simulink model "GFM_NN_closedloop"  (R2025a)
settings: Solver=FixedStepAuto  StartTime=0.0  StopTime=8  FixedStep=1e-6  RelTol=1e-5
PostLoadFcn:
  | , if any(exist('dsrtsu_mdlpostloadfcn', 'file') == [2, 3, 6]), try dsrtsu_mdlpostloadfcn('Execute', bdroot); catch fprintf('Error in PostLoadFcn (dsrtsu_mdlpostloadfcn) for model "%s":\n %s\n', bdroot, lasterr); end, end,
InitFcn:
  | %% ---------sampling time---------
  | fs=10000;
  | Ts = 1/fs; % 1/fs = sampling period;
  | Tsp=Ts;
  | ws=2*pi*fs;
  | Tc = Ts/1;
  | Tch = inf;
  | % Interrupt shift
  | %Tint=0.25e-6;
  | Tint=0.25e-6;
  | %Tint=0;
  | 
  | %% Frequency
  | fsw = 10e3;
  | Tsp = 1 / fsw;
  | % Ts = 1e-6;
  | 
  | %% Grid parameters
  | Vg_LG_RMS = 110;
  | Vg_LL_RMS = Vg_LG_RMS * sqrt(3);
  | f1 = 50;
  | w1 = f1 * 2 * pi;
  | 
  | Lg = 15e-3;
  | Rg = w1 * Lg * 0.05;
  | 
  | %% GFM converter
  | peak_phase_to_earth = sqrt(2)/sqrt(3);
  | SN_GFM = 4e3;
  | PN_GFM = SN_GFM;
  | Vtr_1 = 132;
  | V_base_GFL = Vtr_1*peak_phase_to_earth;
  | I_base_GFL = SN_GFM*peak_phase_to_earth/Vtr_1;
  | 
  | Vs_LL_RMS = Vg_LL_RMS;
  | VDC = 600;
  | 
  | Ls = 3e-3;
  | Rs = w1 * Ls * 0.05;
  | % Rs = 1e-1;
  | Cf = 10e-6;
  | Rf = 1e-3;
  | % Rf = 1;
  | 
  | %% Base values
  | w_Base = 1;
  | %w_Base = 2*pi*f1;
  | V_Base_GFM = sqrt(2) * Vs_LL_RMS / sqrt(3);      % Peak value
  | S_Base_GFM = SN_GFM;
  | I_Base_GFM = sqrt(2) * (S_Base_GFM / 3) / (V_Base_GFM / sqrt(2));     % Peak value
  | Z_Base_GFM = V_Base_GFM / I_Base_GFM;
  | L_Base_GFM = Z_Base_GFM / w_Base;
  | C_Base_GFM = 1 / (w_Base * Z_Base_GFM);
  | 
  | w1_pu = w1 / w_Base;
  | 
  | %% PU values
  | Ls * w1_pu / Z_Base_GFM
  | Ls_pu = Ls / Z_Base_GFM;
  | Lg_pu = Lg / Z_Base_GFM;
  | SCR = 1 / (Lg * w1_pu / Z_Base_GFM)
  | 
  | %% PLL parameters
  | %Kp_PLL = 327.1; %654.3; %32.7;
  | Ki_PLL = 1/0.000013; %1/0.00000325; %1/0.0013;
  | 
  | Kp_SYC = 2;
  | Ki_SYC = 5;
  | 
  | Kp_PQ = 0.1;
  | Ki_PQ = 0.4;
  | 
  | % Kpcc = 5;
  | Kicc = 1/0.01;
  | 
  | %% LPF parameters
  | wp = 2 * pi * 100;
  | wq = 2 * pi * 100;
  | wv = 2 * pi * 100;
  | 
  | %% GFM parameters
  | Pref = 1;
  | kPi = 0.05 * w1_pu;
  | Ra = 0.1;
  | wR = 0.1 * w1_pu;
  | wI = 10 * w1_pu;
  | 
  | kV = 20;
  | kQ = 0.1;
  | 
  | %% Discretization of decoupling
  | s = tf('s');
  | 
  | RV = (Ra*s)/(s+wR);
  | % RV = RV*(wI)/(s+wI);
  | 
  | R1d = c2d(RV , Tsp , 'tustin');
  | dR1num = R1d.Numerator{1};
  | dR1den = R1d.Denominator{1};
  | 
  | %% Discretization of active damping
  | wlpf = 2 * pi * 100;
  | G1st = wlpf / (s + wlpf);
  | G2nd = G1st * G1st;
  | Gc = s * G2nd;
  | Gcd = c2d(Gc , Tsp , 'tustin');
  | 
  | Gcdnum = Gcd.Numerator{1};
  | Gcdden = Gcd.Denominator{1};
  | 
  | %ADC
  | UdcTransdRatio = 25e-3/800;
  | UcaTransdRatio = 25e-3/600;
  | UcbTransdRatio = 25e-3/600;
  | UccTransdRatio = 25e-3/600;
  | UgaTransdRatio = 25e-3/400;
  | UgbTransdRatio = 25e-3/400;
  | UgcTransdRatio = 25e-3/400;
  | 
  | RMeasIa = 220;
  | RMeasIb = 220;
  | RMeasIc = 220;
  | RMeasIdc = 215;
  | RMeasUdc = 237;
  | RMeasUa = 220;
  | RMeasUb = 220;
  | RMeasUc = 220;
  | 
  | LemTurnsIa = 2;
  | LemTurnsIb = 2;
  | LemTurnsIc = 2;
  | 
  | LemTurnsIa1 = 4;
  | LemTurnsIb1 = 4;
  | LemTurnsIc1 = 4;
  | 
  | IaTransdRatio = LemTurnsIa/1000;
  | IbTransdRatio = LemTurnsIb/1000;
  | IcTransdRatio = LemTurnsIc/1000;
  | 
  | IaTransdRatio1 = LemTurnsIa1/1000;
  | IbTransdRatio1 = LemTurnsIb1/1000;
  | IcTransdRatio1 = LemTurnsIc1/1000;
  | 
  | %%
  | %% 1Hz--31Hz  per 1Hz
  | 
  | % degree =5;
  | % K =1;
  | % periods =600;
  | 
  | % PRBS = idinput((2^degree-1), 'prbs');
  | % PRBS = repmat(PRBS,periods + 1,1);
  | % PRBS = K*PRBS;
  | % PRBS_freq =31;
  | 
  | % t_vector=(1/PRBS_freq:1/PRBS_freq:length(PRBS)/PRBS_freq)';
  | % PRBS=[t_vector, PRBS];
  | % stop=t_vector(end);
  | 
  | 
  | %% ====================================================================================================================================================%%
  | %% 10Hz--310Hz  per 10Hz
  | 
  | % degree =5;
  | % K =1.5;
  | % periods =6000;
  | %
  | % PRBS = idinput((2^degree-1), 'prbs');
  | % PRBS = repmat(PRBS,periods + 1,1);
  | % PRBS = K*PRBS;
  | % PRBS_freq =310;
  | %
  | % t_vector=(1/PRBS_freq:1/PRBS_freq:length(PRBS)/PRBS_freq)';
  | % PRBS=[t_vector, PRBS];
  | % stop=t_vector(end);
  | 
  | 
  | %% ====================================================================================================================================================%%
  | %% 100Hz--3100Hz  per 100Hz
  | 
  | % degree =5;
  | % K =2;
  | % periods =10000;
  | %
  | % PRBS = idinput((2^degree-1), 'prbs');
  | % PRBS = repmat(PRBS,periods + 1,1);
  | % PRBS = K*PRBS;
  | % PRBS_freq =3100;
  | %
  | % t_vector=(1/PRBS_freq:1/PRBS_freq:length(PRBS)/PRBS_freq)';
  | % PRBS=[t_vector, PRBS];
  | % stop=t_vector(end);
  | %Kd=1;
  | %wL=0.3*ws;
  | 
  | %L1=4.5e-3;
  | %Tdel=1.5*Ts;
  | %PM=pi/4;%phase margin
  | %wc=(pi/2-PM)/Tdel;%magnitude crossover frequency
  | %Kp=wc*L1;%proportional gain
  | %Ki=wc*Kp/20;%fundamental integrator gain
model workspace (MAT data in the model file):
  W1 = [0.530351698399 -0.46726077795 -0.189978018403 0.581505596638 -0.976636350155 0.285457074642 -0.344555467367 -0.823834598064 0.260987460613 -0.174824804068 0.166140690446 -2.19062757492 ... (5120 elements, 64x80)]
  W2 = [0.0236483272165 -0.12587569654 -3.47338819504 -0.292541116476 -0.164569035172 -0.37011295557 -0.0788608714938 -0.34808665514 -0.0821482911706 0.0780714154243 -0.721733689308 -0.485419809818 ... (1024 elements, 16x64)]
  W3 = [-0.129827529192 0.112917125225 -0.211720749736 0.109386667609 -1.40702748299 -1.11484694481 -0.318361610174 0.218052342534 0.374470740557 -0.190498560667 -0.238774597645 0.996348917484 0.27190181613 -0.264939814806 -0.220842242241 0.382941007614]
  b1 = [-8.9806804657; -10.8322944641; 0.357735663652; -8.11319255829; -12.3089160919; -6.15159845352; -0.239361956716; -10.1425418854; -3.17705559731; -9.53854560852; -2.29398417473; -11.1701593399; -1.7048176527; -9.67482185364; -9.67645168304; -0.294388860464; -2.24801635742; -7.25962114334; -12.5521097183; -6.6342830658; -0.823176324368; 0.253660053015; -8.99686527252; -12.8170499802; -10.1545505524; -2.08569598198; -4.45409345627; -3.44555258751; -10.1237840652; -4.41725730896; -1.93720889091; -11.3758125305; -1.21599435806; -17.1822433472; -2.60073232651; -11.0052156448; -6.07818651199; -9.34351730347; -10.6377429962; 1.69822740555; -9.43974971771; -2.7141919136; -3.19006466866; -11.3538637161; -11.2651071548; -2.94875788689; -1.71119105816; -7.6843419075; -15.207570076; -0.106311887503; -10.9692764282; -0.920050501823; 0.828176736832; -11.2579984665; -9.09425544739; -7.6097574234; -0.587199747562; -5.53113889694; -2.76576495171; -1.6608453989; -10.8241662979; -8.84553050995; -0.99967366457; -11.8896923065]
  b2 = [-0.136206507683; -0.45766967535; -1.54362010956; -0.556495547295; -0.369174063206; -1.49981951714; -1.85871458054; -0.587826907635; -4.87963867188; -1.14077246189; -0.44449698925; -0.9487388134; 2.4190299511; 3.84015583992; -0.180305749178; -0.441644221544]
  b3 = 2.70423817635
  iqrValues = [999.929682567 999.948806394 999.974126382 1163.68199033 1249.86143465 1016.10909761 999.955656405 999.968539404 999.977085124 999.966554003 999.979581889 999.988183479 999.991575713 999.993056679 1000.02967135 1000.00803114 1000.0081017 1210.4487351 1499.93624967 1499.9370729 1406.48598833 937.760144727 1004.26905001 1026.06698255 1138.4066529 1206.84833926 1281.43314966 1372.93379822 1200.77275342 1298.83976016 1490.12450166 1497.42025213 1498.55627365 1498.83428777 1499.24135331 1499.39002656 1499.55488962 1499.65443504 1499.70746847 1499.73165249 1499.74454692 1499.76882354 1499.79135716 1499.80986709 1499.83281542 1499.8484425 1499.8654311 1499.87451238 1499.8928119 1499.9009956 1499.90976565 1499.91746661 1499.92756619 1499.93539792 1499.9414488 1499.94710313 1499.9507773 1499.95615869 1499.96087707 1499.96513792 1499.969596 1499.97293448 1499.97631403 1499.97913361 1499.98180466 1499.98376736 1499.9856365 1499.98732196 1499.98880177 1499.990067 1499.99120073 1499.9922432 1499.9932786 1499.99403762 1499.99470811 1499.99533602 1499.9958744 1499.99636227 1499.99677184 1499.99716187]
  medianValues = [1999.66013382 1999.76293028 1999.73262567 1999.76378275 1999.76361619 1999.77040731 1999.79192245 1999.85691047 1999.87382515 1999.88874694 1999.91524435 1999.91351393 1999.92374826 1999.91295141 1999.89897222 1999.91068089 1999.9210953 1999.9106703 1999.9196212 1999.92798731 1911.70708018 1395.87669838 1499.98470029 1499.98345327 1644.01690443 1805.89164886 1790.23759124 1810.28461467 1819.29782683 1874.70206922 1866.37458572 1829.46040718 1746.52407759 1689.08032976 1634.2809925 1690.42170061 1711.43926014 1714.57960898 1723.90792471 1755.22399993 1766.76731052 1745.61016029 1710.90545293 1744.81369568 1731.87842468 1711.49890061 1691.0235018 1685.21995546 1711.86371385 1706.17582468 1681.04912761 1670.10963643 1649.85367648 1649.94378709 1656.85502029 1681.84492812 1701.45866125 1703.86654039 1702.66606714 1701.58839466 1704.30441478 1719.94997721 1714.50309563 1724.69934828 1742.41991357 1753.39080321 1736.9800895 1742.57116721 1741.00321976 1748.99545485 1735.18183948 1717.61156426 1712.46451329 1713.44210291 1724.88072756 1740.57545678 1739.7916782 1723.53851422 1713.75990069 1700.06444303]
  mu = [-0.108593781339 -0.147308811259 -0.175534555128 -0.136585928467 -0.119784171193 -0.170883245612 -0.185899506459 -0.135931465846 -0.0891217813808 -0.0659545740614 -0.0558679902038 -0.052863332895 -0.0549410539837 -0.0621396876514 -0.0763691039853 -0.102015738859 -0.145826894941 -0.170573714468 -0.166261136131 -0.186454984398 -0.196618728586 -0.0474868984901 0.0493634627812 0.102614249626 0.0637199267366 0.00523193573897 0.00884038490273 -0.00158926451307 -0.0301475501742 -0.0852377475479 -0.0766791293641 -0.054839559592 -0.00114536940186 0.0337163526423 0.0658337208043 0.0239826411048 0.006185576973 0.00390913410424 0.000788598896632 -0.0175293255618 -0.0233896879646 -0.00610338681765 0.0205675702875 -0.00105986382549 0.00664836358885 0.0204692600015 0.0348422547329 0.0376454066957 0.0168967980604 0.0169142911876 0.0308632217189 0.0375731693815 0.0517030134117 0.053006445324 0.0499185751031 0.0347727186848 0.0221713479689 0.0203937937123 0.0208457600537 0.0200998688638 0.0157492005314 0.004180896732 0.00851755521196 0.00304667436411 -0.00686022166667 -0.0127677547474 -0.000952569512195 -0.00260087460801 0.000952261178862 -0.00316737000581 0.00452074549942 0.0133093180822 0.0155023920441 0.0148493657085 0.00767369959059 -0.0025479885453 -0.00170135087108 0.00982238574332 0.0169894429951 0.0259262674216]
  net2 = dlnetwork
  net2.any.Version = 6
  net2.any.LayerGraph = nnet.cnn.LayerGraph
  net2.any.LayerGraph.any.Version = 1
  net2.any.LayerGraph.any.Layers(1) = nnet.cnn.layer.FullyConnectedLayer
  net2.any.LayerGraph.any.Layers(1).any.Version = 3
  net2.any.LayerGraph.any.Layers(1).any.Name = 'dense'
  net2.any.LayerGraph.any.Layers(1).any.InputSize = []
  net2.any.LayerGraph.any.Layers(1).any.OutputSize = 64
  net2.any.LayerGraph.any.Layers(1).any.Weights.Version = 2
  net2.any.LayerGraph.any.Layers(1).any.Weights.Value = [0.530351698399 -0.46726077795 -0.189978018403 0.581505596638 -0.976636350155 0.285457074642 -0.344555467367 -0.823834598064 0.260987460613 -0.174824804068 0.166140690446 -2.19062757492 ... (5120 elements, 64x80)]
  net2.any.LayerGraph.any.Layers(1).any.Weights.LearnRateFactor = 1
  net2.any.LayerGraph.any.Layers(1).any.Weights.L2Factor = 1
  net2.any.LayerGraph.any.Layers(1).any.Weights.Initializer.Version = 1
  net2.any.LayerGraph.any.Layers(1).any.Weights.Initializer.Class = 'nnet.internal.cnn.layer.learnable.initializer.Glorot'
  net2.any.LayerGraph.any.Layers(1).any.Weights.Initializer.ConstructorArguments = {2, 1}
  net2.any.LayerGraph.any.Layers(1).any.Bias.Version = 2
  net2.any.LayerGraph.any.Layers(1).any.Bias.Value = [-8.9806804657; -10.8322944641; 0.357735663652; -8.11319255829; -12.3089160919; -6.15159845352; -0.239361956716; -10.1425418854; -3.17705559731; -9.53854560852; -2.29398417473; -11.1701593399; -1.7048176527; -9.67482185364; -9.67645168304; -0.294388860464; -2.24801635742; -7.25962114334; -12.5521097183; -6.6342830658; -0.823176324368; 0.253660053015; -8.99686527252; -12.8170499802; -10.1545505524; -2.08569598198; -4.45409345627; -3.44555258751; -10.1237840652; -4.41725730896; -1.93720889091; -11.3758125305; -1.21599435806; -17.1822433472; -2.60073232651; -11.0052156448; -6.07818651199; -9.34351730347; -10.6377429962; 1.69822740555; -9.43974971771; -2.7141919136; -3.19006466866; -11.3538637161; -11.2651071548; -2.94875788689; -1.71119105816; -7.6843419075; -15.207570076; -0.106311887503; -10.9692764282; -0.920050501823; 0.828176736832; -11.2579984665; -9.09425544739; -7.6097574234; -0.587199747562; -5.53113889694; -2.76576495171; -1.6608453989; -10.8241662979; -8.84553050995; -0.99967366457; -11.8896923065]
  net2.any.LayerGraph.any.Layers(1).any.Bias.LearnRateFactor = 1
  net2.any.LayerGraph.any.Layers(1).any.Bias.L2Factor = 0
  net2.any.LayerGraph.any.Layers(1).any.Bias.Initializer.Version = 1
  net2.any.LayerGraph.any.Layers(1).any.Bias.Initializer.Class = 'nnet.internal.cnn.layer.learnable.initializer.Zeros'
  net2.any.LayerGraph.any.Layers(1).any.Bias.Initializer.ConstructorArguments = []
  net2.any.LayerGraph.any.Layers(2) = nnet.cnn.layer.ReLULayer
  net2.any.LayerGraph.any.Layers(2).any.Version = 1
  net2.any.LayerGraph.any.Layers(2).any.Name = 'dense_relu'
  net2.any.LayerGraph.any.Layers(3) = nnet.cnn.layer.FullyConnectedLayer
  net2.any.LayerGraph.any.Layers(3).any.Version = 3
  net2.any.LayerGraph.any.Layers(3).any.Name = 'dense_1'
  net2.any.LayerGraph.any.Layers(3).any.InputSize = []
  net2.any.LayerGraph.any.Layers(3).any.OutputSize = 16
  net2.any.LayerGraph.any.Layers(3).any.Weights.Version = 2
  net2.any.LayerGraph.any.Layers(3).any.Weights.Value = [0.0236483272165 -0.12587569654 -3.47338819504 -0.292541116476 -0.164569035172 -0.37011295557 -0.0788608714938 -0.34808665514 -0.0821482911706 0.0780714154243 -0.721733689308 -0.485419809818 ... (1024 elements, 16x64)]
  net2.any.LayerGraph.any.Layers(3).any.Weights.LearnRateFactor = 1
  net2.any.LayerGraph.any.Layers(3).any.Weights.L2Factor = 1
  net2.any.LayerGraph.any.Layers(3).any.Weights.Initializer.Version = 1
  net2.any.LayerGraph.any.Layers(3).any.Weights.Initializer.Class = 'nnet.internal.cnn.layer.learnable.initializer.Glorot'
  net2.any.LayerGraph.any.Layers(3).any.Weights.Initializer.ConstructorArguments = {2, 1}
  net2.any.LayerGraph.any.Layers(3).any.Bias.Version = 2
  net2.any.LayerGraph.any.Layers(3).any.Bias.Value = [-0.136206507683; -0.45766967535; -1.54362010956; -0.556495547295; -0.369174063206; -1.49981951714; -1.85871458054; -0.587826907635; -4.87963867188; -1.14077246189; -0.44449698925; -0.9487388134; 2.4190299511; 3.84015583992; -0.180305749178; -0.441644221544]
  net2.any.LayerGraph.any.Layers(3).any.Bias.LearnRateFactor = 1
  net2.any.LayerGraph.any.Layers(3).any.Bias.L2Factor = 0
  net2.any.LayerGraph.any.Layers(3).any.Bias.Initializer.Version = 1
  net2.any.LayerGraph.any.Layers(3).any.Bias.Initializer.Class = 'nnet.internal.cnn.layer.learnable.initializer.Zeros'
  net2.any.LayerGraph.any.Layers(3).any.Bias.Initializer.ConstructorArguments = []
  net2.any.LayerGraph.any.Layers(4) = nnet.cnn.layer.ReLULayer
  net2.any.LayerGraph.any.Layers(4).any.Version = 1
  net2.any.LayerGraph.any.Layers(4).any.Name = 'dense_1_relu'
  net2.any.LayerGraph.any.Layers(5) = nnet.cnn.layer.FullyConnectedLayer
  net2.any.LayerGraph.any.Layers(5).any.Version = 3
  net2.any.LayerGraph.any.Layers(5).any.Name = 'dense_2'
  net2.any.LayerGraph.any.Layers(5).any.InputSize = []
  net2.any.LayerGraph.any.Layers(5).any.OutputSize = 1
  net2.any.LayerGraph.any.Layers(5).any.Weights.Version = 2
  net2.any.LayerGraph.any.Layers(5).any.Weights.Value = [-0.129827529192 0.112917125225 -0.211720749736 0.109386667609 -1.40702748299 -1.11484694481 -0.318361610174 0.218052342534 0.374470740557 -0.190498560667 -0.238774597645 0.996348917484 0.27190181613 -0.264939814806 -0.220842242241 0.382941007614]
  net2.any.LayerGraph.any.Layers(5).any.Weights.LearnRateFactor = 1
  net2.any.LayerGraph.any.Layers(5).any.Weights.L2Factor = 1
  net2.any.LayerGraph.any.Layers(5).any.Weights.Initializer.Version = 1
  net2.any.LayerGraph.any.Layers(5).any.Weights.Initializer.Class = 'nnet.internal.cnn.layer.learnable.initializer.Glorot'
  net2.any.LayerGraph.any.Layers(5).any.Weights.Initializer.ConstructorArguments = {2, 1}
  net2.any.LayerGraph.any.Layers(5).any.Bias.Version = 2
  net2.any.LayerGraph.any.Layers(5).any.Bias.Value = 2.70423817635
  net2.any.LayerGraph.any.Layers(5).any.Bias.LearnRateFactor = 1
  net2.any.LayerGraph.any.Layers(5).any.Bias.L2Factor = 0
  net2.any.LayerGraph.any.Layers(5).any.Bias.Initializer.Version = 1
  net2.any.LayerGraph.any.Layers(5).any.Bias.Initializer.Class = 'nnet.internal.cnn.layer.learnable.initializer.Zeros'
  net2.any.LayerGraph.any.Layers(5).any.Bias.Initializer.ConstructorArguments = []
  net2.any.LayerGraph.any.Layers(6) = nnet.cnn.layer.SigmoidLayer
  net2.any.LayerGraph.any.Layers(6).Name = 'dense_2_sigmoid'
  net2.any.LayerGraph.any.Layers(6).Description = 'sigmoid'
  net2.any.LayerGraph.any.Layers(6).Type = 'Sigmoid'
  net2.any.LayerGraph.any.Layers(6).PrivateNumStates = 0
  net2.any.LayerGraph.any.Layers(7) = nnet.cnn.layer.FeatureInputLayer
  net2.any.LayerGraph.any.Layers(7).any.Version = 2
  net2.any.LayerGraph.any.Layers(7).any.Name = 'input'
  net2.any.LayerGraph.any.Layers(7).any.InputSize = 80
  net2.any.LayerGraph.any.Layers(7).any.Normalization = []
  net2.any.LayerGraph.any.Layers(7).any.NormalizationDimension = 'auto'
  net2.any.LayerGraph.any.Layers(7).any.SplitComplexInputs = 0
  net2.any.LayerGraph.any.Connections = table
  net2.any.LayerGraph.any.Connections.data = {{'dense'; 'dense_relu'; 'dense_1'; 'dense_1_relu'; 'dense_2'; 'input'}, {'dense_relu'; 'dense_1'; 'dense_1_relu'; 'dense_2'; 'dense_2_sigmoid'; 'dense'}}
  net2.any.LayerGraph.any.Connections.ndims = 2
  net2.any.LayerGraph.any.Connections.nrows = 6
  net2.any.LayerGraph.any.Connections.nvars = 2
  net2.any.LayerGraph.any.Connections.varnames = {'Source', 'Destination'}
  net2.any.LayerGraph.any.Connections.props.CustomProps = struct()
  net2.any.LayerGraph.any.Connections.props.VariableCustomProps = struct()
  net2.any.LayerGraph.any.Connections.props.versionSavedFrom = 5
  net2.any.LayerGraph.any.Connections.props.minCompatibleVersion = 1
  net2.any.LayerGraph.any.Connections.props.incompatibilityMsg = ''
  net2.any.LayerGraph.any.Connections.props.VersionSavedFrom = 5
  net2.any.LayerGraph.any.Connections.props.useVariableNamesOriginal = 0
  net2.any.LayerGraph.any.Connections.props.useVariableNames2048 = 0
  net2.any.LayerGraph.any.Connections.props.useDimensionNamesOriginal = 0
  net2.any.LayerGraph.any.Connections.props.useDimensionNames2048 = 0
  net2.any.LayerGraph.any.Connections.props.Description = ''
  net2.any.LayerGraph.any.Connections.props.VariableNamesOriginal = {}
  net2.any.LayerGraph.any.Connections.props.VariableNames2048 = {}
  net2.any.LayerGraph.any.Connections.props.DimensionNames = {'Row', 'Variables'}
  net2.any.LayerGraph.any.Connections.props.DimensionNamesOriginal = {}
  net2.any.LayerGraph.any.Connections.props.DimensionNames2048 = {}
  net2.any.LayerGraph.any.Connections.props.UserData = []
  net2.any.LayerGraph.any.Connections.props.VariableDescriptions = {}
  net2.any.LayerGraph.any.Connections.props.VariableUnits = {}
  net2.any.LayerGraph.any.Connections.props.VariableContinuity = {}
  net2.any.Initialized = 1
  net2.any.SerializedQuantizationInfo.version = 1
  net2.any.SerializedQuantizationInfo.data = containers.Map
  net2.any.SerializedQuantizationInfo.data.serialization.keys = {}
  net2.any.SerializedQuantizationInfo.data.serialization.values = {}
  net2.any.SerializedQuantizationInfo.data.serialization.uniformity = 0
  net2.any.SerializedQuantizationInfo.data.serialization.keyType = 'char'
  net2.any.SerializedQuantizationInfo.data.serialization.valueType = 'any'
  net2.any.ExampleInputs = {}
  net2.any.OutputNames = {'dense_2_sigmoid'}
  net2.any.ExternalOutputNames = []
  net2.any.ExternalInputNames = []
  net2.any.RetainCustomInputNames = 1
  net2.any.RetainCustomOutputNames = 1
  sigma = [0.7187830922 0.834238393845 0.919900139685 0.688758980318 0.599693957155 0.858339742411 0.965167977116 0.792700626358 0.681503940515 0.658236278259 0.655707879722 0.655775233832 0.655036132409 0.653768282287 0.655510425327 0.67348507997 0.743792493648 0.73016256957 0.614179141359 0.623947550127 0.778535364401 0.909651097701 0.727286163536 0.70671836313 0.777236577422 0.769324914099 0.595403383999 0.540696552337 0.662939303255 0.648997635583 0.57561594459 0.568737612456 0.565218359851 0.569606620826 0.576583341372 0.584885124684 0.593551108815 0.59229435351 0.581309320924 0.576350786773 0.57666876863 0.570581319292 0.560793531842 0.560694006623 0.566916161302 0.566088166849 0.561418971234 0.56235821277 0.568335821314 0.576673692472 0.583008390922 0.582581690634 0.580788739269 0.577441504306 0.574909719909 0.571474255548 0.571501878774 0.572126163619 0.570647345246 0.572631759715 0.579607159686 0.582036558737 0.57906813539 0.576631229054 0.573073934433 0.57205576392 0.574344093466 0.57063072067 0.563735477399 0.559835697201 0.564270823814 0.573365736852 0.574551937463 0.572999012788 0.571170204611 0.571628429237 0.571978711484 0.571091952605 0.56861071165 0.569309579382]
undefined symbols (not defined in the file): DiscIntNeverNeededParam
libraries: spsSeriesRLCBranchLib x18, spsCurrentMeasurementLib x9, simulink x6, spsVoltageMeasurementLib x6, simulink_extras x4, spsGroundLib x4, plecslib_extras x2, deeplib x1, spsDCVoltageSourceLib x1, spsThreePhaseProgrammableVoltageSourceLib x1, spsTwoLevelConverterLib x1, spspowerguiLib x1
(part 1 of 3)
settings Model: DSRTSU_INTERNAL_RTI_VER=520  DSRTSU_INTERNAL_RTI_TYPE=rti1007  DSRTSU_INTERNAL_RTIFPGA=110  RTICANMMDATA=struct('GeneralSetupData',struct('modelroot',['C:\Users\Lab User\Desktop\Exp_2022_0406\Matlab'],'generalsettings',struct('filesettings',struct('destfolder',struct('Name','RTICANMM_FILES','Check',1),'buildfolder',struct('Name','.','Check',1),'AbsDestfolder',struct('Name',['C:\Users\Lab User\Desktop\Exp_2022_0406\Matlab\RTICANMM_FILES']),'AbsBuildfolder',struct('Name',['C:\Users\Lab User\Desktop\Exp_2022_0406\Matlab']))),'options',struct('addpaths',1,'rmpaths',1,'addtrcexclusion',logical(1),'cannavigator',struct('checkmonitoring',0),'show_usrtrc',0,'use_usrtrc',0),'advanced',struct('options',[1 1 1 1 1 1 1 1 1 1 1 1 1 1 1 1 1 1 1 1 1 1 1 1 1 1 1 1 1 1 1 1 1 1 1 1 1 1 1 1 1 1 1 1 1 1 1 1 1 1 1 1 1 1 1 1 1 1 1 1 1 1 1 1 1 1 1 1 1 1 1 1 1 1 1 1 1 1 1 1 1 1 1 1 1 1 1 1 1 1 1 1 1 1 1 1 1 1 1 1]),'MPSetup',{{}},'modelname','newp_fzha_20220406_2017b','block','newp_fzha_20220406_2017b'))  DSRTSU_INTERNAL_RTIFLEXRAYCONFIG=110  Creator=xwa  LastModifiedBy=yangwu
settings SolverCC: ZeroCrossAlgorithm=Adaptive  AutoInsertRateTranBlk=on
settings DataIOCC: LimitDataPoints=on  SaveFormat=Array  SignalLoggingSaveFormat=ModelDataLogs  ReturnWorkspaceOutputs=off
settings OptimizationCC: BlockReduction=off  OptimizeBlockIOStorage=off  BufferReuse=off  ReuseModelBlockBuffer=off  GlobalBufferReuse=off  ExpressionFolding=off  ExpressionDepthLimit=2147483647.0  LocalBlockOutputs=off  LifeSpan=inf  OptimizeDataStoreBuffers=off  BusAssignmentInplaceUpdate=off
settings DebuggingCC: UnderspecifiedInitializationDetection=Classic  MergeDetectMultiDrivingBlocksExec=none  IgnoredZcDiagnostic=none  SolverPrmCheckMsg=warning  FcnCallInpInsideContextMsg=warning  UnconnectedInputMsg=warning  UnconnectedOutputMsg=warning  UnconnectedLineMsg=warning  StateNameClashWarn=warning  SFUnexpectedBacktrackingDiag=warning  SFNoUnconditionalDefaultTransitionDiag=warning  SFExecutionAtInitializationDiag=none  ArithmeticOperatorsInVariantConditions=warning
settings HardwareCC: ProdBitPerPointer=32.0  ProdBitPerSizeT=32.0  ProdBitPerPtrDiffT=32.0  ProdLargestAtomicInteger=Integer  ProdEndianess=BigEndian  ProdWordSize=32.0  ProdHWDeviceType=Custom Processor->Custom  TargetIntDivRoundTo=Zero  TargetEndianess=BigEndian  TargetHWDeviceType=Custom Processor->Custom
settings ModelReferenceCC: EnableRefExpFcnMdlSchedulingChecks=on  PropagateSignalLabelsOutOfModel=off
settings SFSimCC: SimUseLocalCustomCode=off  MATLABDynamicMemAlloc=off  CustomCodeUndefinedFunction=UseInterfaceOnly
settings RTWCC: SystemTargetFile=rti1007.tlc  MakeCommand=make_rti  TemplateMakefile=rti1007.tmf  RTWUseLocalCustomCode=off  GPUComputeCapability=3.5  Description=dSPACE DS1007 Hardware Platform
settings CodeAppCC: StateflowObjectComments=on
settings STFCustomTargetCC: SystemTargetFile=rti1007.tlc  MultiwordLength=2048.0  DynamicStringBufferSize=256.0  ParMdlRefBuildCompliant=on  GRTInterface=off  EnableRealTimeTesting=on  TaskModeNonUI=LOW_JITTER  AssertionMode=OFF  TRCGenerateDerivatives=off  ExecutionMode=real-time  LoadAfterBuild=on  TRCGenerateVirtualBlocks=on  LoadApplNonUI=ON  RTICfgSetVer=520.0  CCompilerOptimizationOptsPopup_=Default  EnableRealTimeTestingNonUI=ON  TRCGenerateParamValues=off  LoadToFlash=off  CCompilerOptimizationOptsNonUI=USE_DEFAULT  TaskMode=Low jitter, low latency tasks  BoardNameNonUI=ds1007  TRCGenerateStates=off  TRCGenerateLabels=on  TimeScaleFactorNonUI=OPTION_DISABLED  TimeScaleFactor=1.0  ExecutionModeNonUI=RTSIM  InitialSimState=RUN  AllowReservedHostServiceNums=off  BoardName=ds1007  TRCIsOmitVdOn=off  TRCOnlyGlobals=off  PlatformSelectionPopup=Platform Name  NetworkClientNonUI=OPTION_DISABLED
settings GRTTargetCC: ExtModeMexFile=noextcomm  TargetLangStandard=C89/C90 (ANSI)  CompOptLevelCompliant=off  ConcurrentExecutionCompliant=off  CombineOutputUpdateFcns=off  MatFileLogging=off  CPPClassGenCompliant=off  UseToolchainInfoCompliant=off
settings ConfigComp: CovMetricSettings=dw  CovSaveCumulativeToWorkspaceVar=on  CovSaveSingleToWorkspaceVar=on  CovExternalEMLEnable=off

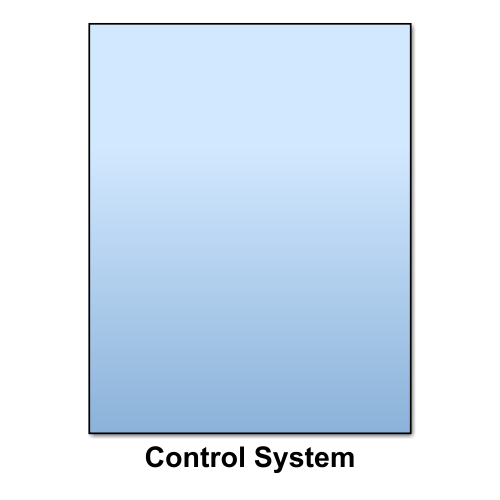
[thumbnail: Simulink's stored preview of the top-level diagram]
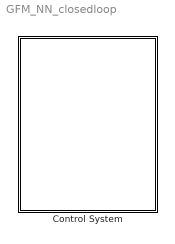
== system GFM_NN_closedloop ==
  Control System : Subsystem
